simulink model "Comparacion_simulink_ej7"  (R2020a)
settings: Solver=ode45  StartTime=0.0  StopTime=10  MaxStep=1e-4  RelTol=1e-3
values from neighbouring files (symbols this model uses):
  kp = k(indice, 1)    [Ejercicio1_parametros.m]
undefined symbols (not defined in the file or in its folder): kdr, kir, sigbuilder_block
libraries: simulink x2
settings Model: Creator=juan  LastModifiedBy=juan

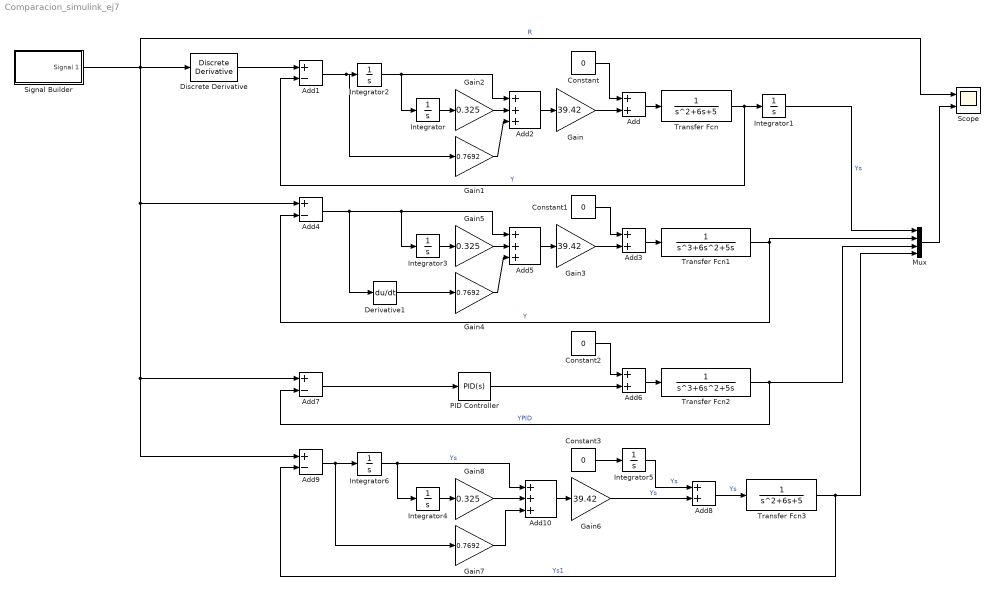
== system Comparacion_simulink_ej7 ==
  Add{,3,6,8} (4 alike) : Sum
  Add{1,4,7,9} (4 alike) : Sum  Inputs=+-
  Add10 : Sum  Inputs=+++
  Add2 : Sum  Inputs=+++
  Add5 : Sum  Inputs=+++
  Constant{,1..3} (4 alike) : Constant  Value=0
  Derivative1 : Derivative  CoefficientInTFapproximation=0.01
  Discrete Derivative : simulink/Discrete/Discrete Derivative  gainval=1.0  ICPrevScaledInput=0.0  OutMin=[]  OutMax=[]  OutDataType=fixdt(1, 16)  OutScaling=2^-10  DoSatur=off
  Gain : Gain  Gain=39.42
  Gain1 : Gain  Gain=0.7692
  Gain2 : Gain  Gain=0.325
  Gain3 : Gain  Gain=39.42
  Gain4 : Gain  Gain=0.7692
  Gain5 : Gain  Gain=0.325
  Gain6 : Gain  Gain=39.42
  Gain7 : Gain  Gain=0.7692
  Gain8 : Gain  Gain=0.325
  Integrator{,1..6} (7 alike) : Integrator
  Mux : Mux
  PID Controller : simulink/Continuous/PID Controller  Controller=PID  Form=Parallel  TimeDomain=Continuous-time  UseExternalTs=off  SampleTime=-1  IntegratorMethod=Forward Euler  FilterMethod=Forward Euler  ControllerParametersSource=internal  P=kp  I=kp*kir  D=kp*kdr  UseFilter=on  N=100  TunerSelectOption=Transfer Function Based (PID Tuner App)  InitialConditionSource=internal  InitialConditionForIntegrator=0  InitialConditionForFilter=0  DifferentiatorICPrevScaledInput=0  ExternalReset=none  TrackingMode=off  Kt=1  LimitOutput=off  UpperSaturationLimit=inf  LowerSaturationLimit=-inf  LinearizeAsGain=on  AntiWindupMode=none  Kb=1  POutMin=[]  POutMax=[]  IOutMin=[]  IOutMax=[]  DOutMin=[]  DOutMax=[]  NOutMin=[]  NOutMax=[]  SumOutMin=[]  SumOutMax=[]  SaturationOutMin=[]  SaturationOutMax=[]  PParamMin=[]  PParamMax=[]  IParamMin=[]  IParamMax=[]  DParamMin=[]  DParamMax=[]  NParamMin=[]  NParamMax=[]  KbParamMin=[]  KbParamMax=[]  KtParamMin=[]  KtParamMax=[]  KbOutMin=[]  KbOutMax=[]  KtOutMin=[]  KtOutMax=[]  IntegratorOutMin=[]  IntegratorOutMax=[]  FilterOutMin=[]  FilterOutMax=[]  SumI1OutMin=[]  SumI1OutMax=[]  SumI2OutMin=[]  SumI2OutMax=[]  SumI3OutMin=[]  SumI3OutMax=[]  SumI4OutMin=[]  SumI4OutMax=[]  SumDOutMin=[]  SumDOutMax=[]  DifferentiatorOutMin=[]  DifferentiatorOutMax=[]  FilterDiffOutCoefMin=[]  FilterDiffOutCoefMax=[]  ReciprocalOutMin=[]  ReciprocalOutMax=[]  SumDenOutMin=[]  SumDenOutMax=[]  SumNumOutMin=[]  SumNumOutMax=[]  DivideOutMin=[]  DivideOutMax=[]  UdiffTsProdOutMin=[]  UdiffTsProdOutMax=[]  NTsProdOutMin=[]  NTsProdOutMax=[]  UintegralTsProdOutMin=[]  UintegralTsProdOutMax=[]  UngainTsProdOutMin=[]  UngainTsProdOutMax=[]  IntegratorContinuousStateAttributes=''  IntegratorStateMustResolveToSignalObject=off  IntegratorRTWStateStorageClass=Auto  FilterContinuousStateAttributes=''  FilterStateMustResolveToSignalObject=off  FilterRTWStateStorageClass=Auto  ParallelPVariant=InternalParameters  IdealPVariant=Disabled  IVariant=InternalParameters  DVariant=InternalParameters  IntegratorVariant=Continuous  SatVariant=Disabled  AWVariant=Passthrough  PCopyVariant=Disabled  TRVariant=Disabled  FdbkBlocksVariant=Forward  IdealPFdbkVariant=Disabled  SatFdbkVariant=Disabled  DerivativeFilterVariant=ContFilter  NVariant=InternalParameters  NCopyVariant=Disabled  FilterICVariant=InternalICsFilter  IntegratorICVariant=InternalICs  ExternalResetVariant=Disabled  TRSumVariant=Passthrough  SumFdbkVariant=Disabled  SumVariant=Sum_PID  TsampFilterVariant=InternalTs  TsampNgainVariant=Passthrough  TsampIntegralVariant=Passthrough
  Scope : Scope  NumInputPorts=2
  Signal Builder : Subsystem  Tag=STV Subsys  LoadFcn=sigbuilder_block('load');  StartFcn=sigbuilder_block('start');  StopFcn=sigbuilder_block('stop');  ClipboardFcn=sigbuilder_block('clipboard');  mask(Sigbuilder block){tuvar=[0:10]}
      mask help: Simulink:masks:SigbuilderBlock_MD
      mask init:
      | if ~strcmp(get_param(bdroot(gcbh),'SimulationStatus'),'stopped') tuvar = sigbuilder_block('maskInit'); end
      settings: CopyFcn=sigbuilder_block('copy');  DeleteFcn=sigbuilder_block('delete');  ModelCloseFcn=sigbuilder_block('modelClose');  PreSaveFcn=sigbuilder_block('preSave');  PauseFcn=sigbuilder_block('pause');  ContinueFcn=sigbuilder_block('continue');  NameChangeFcn=sigbuilder_block('namechange');  OpenFcn=sigbuilder_block('open',[0 22.5 1024.5 495.75 ]);  CloseFcn=sigbuilder_block('close');
      mask Display: plot(0, 0, 100, 100,[2, 2, 32, 32, 2], [68, 8, 8, 68, 68],[32, 2], [38, 38], [32, 19, 2],[53, 60, 44], [32, 17, 17, 2],[16, 16, 31, 31]);txt = getActiveGroup(gcbh);text(2, 100, txt,'verticalAlignment', 'top');
  Transfer Fcn : TransferFcn  Denominator=[1 6 5 ]
  Transfer Fcn1 : TransferFcn  Denominator=[1 6 5 0]
  Transfer Fcn2 : TransferFcn  Denominator=[1 6 5 0]
  Transfer Fcn3 : TransferFcn  Denominator=[1 6 5 ]
  wires:
  Add/1 -> Transfer Fcn/1
  Constant/1 -> Add/1
  Add2/1 -> Gain/1
  Gain1/1 -> Add2/3
  Gain2/1 -> Add2/2
  Transfer Fcn/1 -> Integrator1/1, Add1/2  "Y"
  Integrator/1 -> Gain2/1
  Add1/1 -> Gain1/1, Integrator2/1
  Gain/1 -> Add/2
  Integrator1/1 -> Mux/1  "Ys"
  Integrator2/1 -> Integrator/1, Add2/1
  Gain3/1 -> Add3/2
  Gain4/1 -> Add5/3
  Add4/1 -> Integrator3/1, Add5/1, Derivative1/1
  Integrator3/1 -> Gain5/1
  Transfer Fcn1/1 -> Mux/2, Add4/2  "Y"
  Gain5/1 -> Add5/2
  Add3/1 -> Transfer Fcn1/1
  Add5/1 -> Gain3/1
  Constant1/1 -> Add3/1
  Mux/1 -> Scope/2
  Constant2/1 -> Add6/1
  Add6/1 -> Transfer Fcn2/1
  PID Controller/1 -> Add6/2
  Transfer Fcn2/1 -> Mux/3, Add7/2  "YPID"
  Add7/1 -> PID Controller/1
  Discrete Derivative/1 -> Add1/1
  Derivative1/1 -> Gain4/1
  Add9/1 -> Integrator6/1, Gain7/1
  Signal Builder/1(Signal 1) -> Add4/1, Add9/1, Add7/1, Scope/1, Discrete Derivative/1  "R"
  Gain8/1 -> Add10/2
  Gain7/1 -> Add10/3
  Integrator4/1 -> Gain8/1
  Constant3/1 -> Integrator5/1
  Add10/1 -> Gain6/1
  Add8/1 -> Transfer Fcn3/1  "Ys"
  Integrator5/1 -> Add8/1  "Ys"
  Gain6/1 -> Add8/2  "Ys"
  Integrator6/1 -> Integrator4/1, Add10/1  "Ys"
  Transfer Fcn3/1 -> Mux/4, Add9/2  "Ys1"

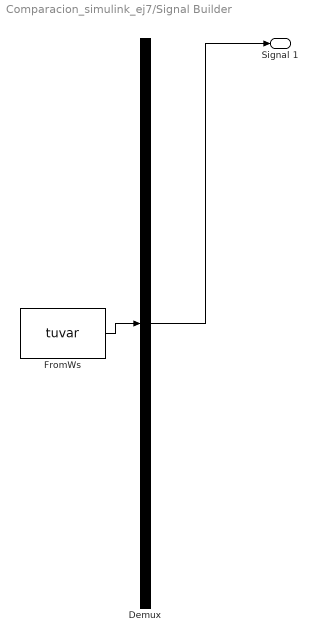
== system Comparacion_simulink_ej7/Signal Builder ==
  Demux : Demux  Tag=STV Demux  Outputs=1
      settings: DisplayOption=none
  FromWs : FromWorkspace  Tag=STV FromWs  VariableName=tuvar
      SigBuilderData=|
      | common.afterFinalStr = 'Extrapolate'
      | common.sampleTime = 0
      | dataSet.timeRange = [0 10]
      | dataSet.name = 'Group 1'
      | sbobj.Groups.Name = 'Group 1'
      | sbobj.Groups.Signals.Name = 'Signal 1'
      | sbobj.Groups.Signals.XData = [0 1 1 6 10]
      | sbobj.Groups.Signals.YData = [0 0 1 1 1]
  Signal 1 : Outport  Tag=STV Outport
  wires:
  Demux/1 -> Signal 1/1
  FromWs/1 -> Demux/1
